simulink model "lab3_sim_2018"  (R2018b)
settings: Solver=FixedStepAuto  StartTime=0.0  StopTime=100  FixedStep=1e-4  RelTol=1e-3
values from neighbouring files (symbols this model uses):
  A = [0, 1, 0, 0;-ks/ms, -T/ms, ks/ms, 0;0, 0, 0, 1;ks/mp, T/mp, -(ks + kp)/mp, -cp/mp]    [lab3_Task_4.m]    (also in lab3_Task_5.m = [0, 1, 0, 0; lab3_Task_5_old.m = [0, 1, 0, 0)
  Ash = [0, 1, 0, 0 ... (first row only)    [getUpdatedModel.m]    (also in lab3_Task_5.m; lab3_Task_5_old.m = [0, 0, 0, 0; lab_3_model_uncertainity.m)
  B = [0, 0; 0, 0; 0, 0; kp/mp, cp/mp]    [lab3_Task_4.m]    (also in lab3_Task_5.m = [0,0,0,0; lab3_Task_5_old.m = [0,0,0,0)
  Bsh = [0,0,0,0 ... (first row only)    [getUpdatedModel.m]    (also in lab3_Task_5.m; lab3_Task_5_old.m = [0,0,-1/cz,-1/cz; lab_3_model_uncertainity.m)
  C = [1, 0, 0, 0]    [lab3_Task_4.m]    (also in lab3_Task_5.m = [1, 0, 0, 0; lab3_Task_5_old.m = [1, 0, 0, 0)
  Csh = [0, 1, 0, 0 ... (first row only)    [lab3_Task_5.m]    (also in lab3_Task_5_old.m = [1,0, 0, 0; lab_3_model_uncertainity.m = [1,0, 0, 0)
  D = 0    [lab3_Task_4.m]    (also in lab3_Task_5.m = zeros(2,4); lab3_Task_5_old.m = zeros(2,4))
  Dsh = zeros(2,4)    [lab3_Task_5.m]    (also in lab3_Task_5_old.m = zeros(4,4); lab_3_model_uncertainity.m = zeros(4,4))
undefined symbols (not defined in the file or in its folder): sigbuilder_block
settings Model: Creator=Hp  LastModifiedBy=anirv
settings DataIOCC: ReturnWorkspaceOutputs=on

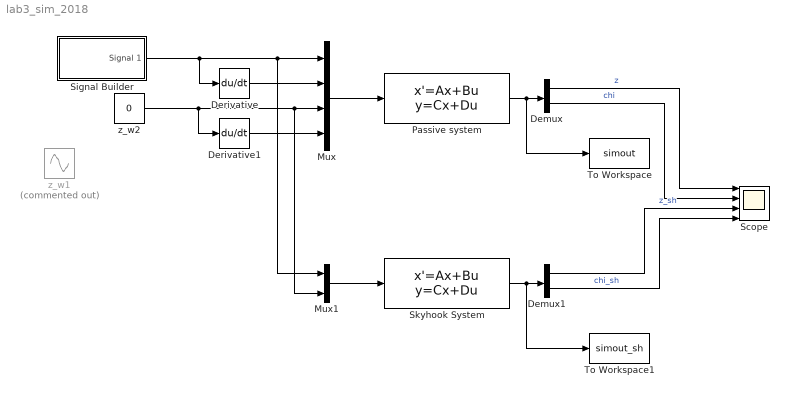
== system lab3_sim_2018 ==
  Demux : Demux  Outputs=2
  Demux1 : Demux  Outputs=2
  Derivative : Derivative
  Derivative1 : Derivative
  Mux : Mux
  Mux1 : Mux  Inputs=2
  Passive system : StateSpace  A=A  B=B  C=C  D=D  InitialCondition=0  ContinuousStateAttributes={'zs','zs_dot','chi','chi_dot'}
  Scope : Scope  NumInputPorts=4
  Signal Builder : Subsystem  Tag=STV Subsys  LoadFcn=sigbuilder_block('load');  StartFcn=sigbuilder_block('start');  StopFcn=sigbuilder_block('stop');  ClipboardFcn=sigbuilder_block('clipboard');  mask(Sigbuilder block){tuvar=[0:10]}
      mask help: Simulink:masks:SigbuilderBlock_MD
      mask init:
      | if ~strcmp(get_param(bdroot(gcbh),'SimulationStatus'),'stopped') tuvar = sigbuilder_block('maskInit'); end
      settings: CopyFcn=sigbuilder_block('copy');  DeleteFcn=sigbuilder_block('delete');  ModelCloseFcn=sigbuilder_block('modelClose');  PreSaveFcn=sigbuilder_block('preSave');  PauseFcn=sigbuilder_block('pause');  ContinueFcn=sigbuilder_block('continue');  NameChangeFcn=sigbuilder_block('namechange');  OpenFcn=sigbuilder_block('open',[5.4 30 1141.2 522.6 ]);  CloseFcn=sigbuilder_block('close');
      mask Display: plot(0, 0, 100, 100,[2, 2, 32, 32, 2], [68, 8, 8, 68, 68],[32, 2], [38, 38], [32, 19, 2],[53, 60, 44], [32, 17, 17, 2],[16, 16, 31, 31]);txt = getActiveGroup(gcbh);text(2, 100, txt,'verticalAlignment', 'top');
  Skyhook System : StateSpace  A=Ash  B=Bsh  C=Csh  D=Dsh  InitialCondition=0  ContinuousStateAttributes={'zs','zs_dot','chi','chi_dot'}
  To Workspace : ToWorkspace  VariableName=simout  SaveFormat=Timeseries  SampleTime=-1
  To Workspace1 : ToWorkspace  VariableName=simout_sh  SaveFormat=Timeseries  SampleTime=-1
  z_w1 : Sin  Commented=on  Amplitude=0.01  Frequency=6.28  SampleTime=0
  z_w2 : Constant  Value=0
  wires:
  Derivative/1 -> Mux/2
  Mux/1 -> Passive system/1
  Signal Builder/1(Signal 1) -> Derivative/1, Mux1/1, Mux/1
  z_w2/1 -> Derivative1/1, Mux1/2, Mux/3
  Derivative1/1 -> Mux/4
  Passive system/1 -> To Workspace/1, Demux/1
  Demux/1 -> Scope/1  "z"
  Demux/2 -> Scope/2  "chi"
  Skyhook System/1 -> To Workspace1/1, Demux1/1
  Mux1/1 -> Skyhook System/1
  Demux1/1 -> Scope/3  "z_sh"
  Demux1/2 -> Scope/4  "chi_sh"

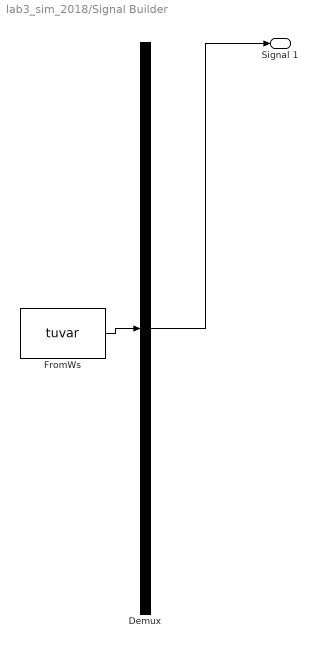
== system lab3_sim_2018/Signal Builder ==
  Demux : Demux  Tag=STV Demux  Outputs=1
  FromWs : FromWorkspace  Tag=STV FromWs  VariableName=tuvar  SampleTime=0
      SigBuilderData=|
      | common.afterFinalStr = 'Extrapolate'
      | common.sampleTime = 0
      | dataSet.timeRange = [0 60]
      | dataSet.name = 'Group 1'
      | sbobj.Groups.Name = 'Group 1'
      | sbobj.Groups.Signals.Name = 'Signal 1'
      | sbobj.Groups.Signals.XData = [0 33.3 33.3 60]
      | sbobj.Groups.Signals.YData = [0.03 0.03 0 0]
      | sbobj.Groups.TimeRange = [0 60]
  Signal 1 : Outport  Tag=STV Outport  VectorParamsAs1DForOutWhenUnconnected=on
  wires:
  Demux/1 -> Signal 1/1
  FromWs/1 -> Demux/1
